simulink library "MofNFilterBlock"  (R2018b)
settings: Solver=VariableStepAuto  StartTime=0.0  StopTime=10.0  RelTol=1e-3
undefined symbols (not defined in the file): filter_M_down, filter_M_up, filter_N
libraries: simulink x1
settings Model: Creator=BI28030  LastModifiedBy=BI28030

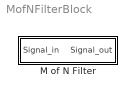
== system MofNFilterBlock ==
  M of N Filter : Subsystem  mask{num_samples=filter_N, num_upgrade=filter_M_up, num_downgrade=filter_M_down}
      mask prompts: num_samples "Number of Samples (N)"; num_upgrade "Number for Upgrade (M)"; num_downgrade "Number for Downgrade (M)"

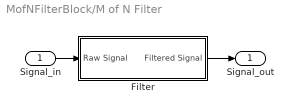
== system MofNFilterBlock/M of N Filter ==
  Signal_in : Inport
  Filter : Subsystem  mask(Alert Filter){num_samples_signal=num_samples, threshold_signal=num_upgrade, threshold_downgrade=num_downgrade}
      mask prompts: num_samples_signal "Number of Raw Signal Samples"; threshold_signal "Number of Positives for Signal upgrade"; threshold_downgrade "Number of Negatives for Downgrade"
      mask help: Filters stream of raw alerts to compensate for surveillance noise.
  Signal_out : Outport
  wires:
  Filter/1(Filtered Signal) -> Signal_out/1
  Signal_in/1 -> Filter/1(Raw Signal)

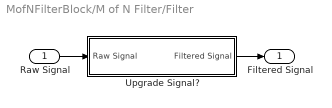
== system MofNFilterBlock/M of N Filter/Filter ==
  Raw Signal : Inport
  Upgrade Signal? : Subsystem  TreatAsAtomicUnit=on
  Filtered Signal : Outport
  wires:
  Upgrade Signal?/1(Filtered Signal) -> Filtered Signal/1
  Raw Signal/1 -> Upgrade Signal?/1(Raw Signal)

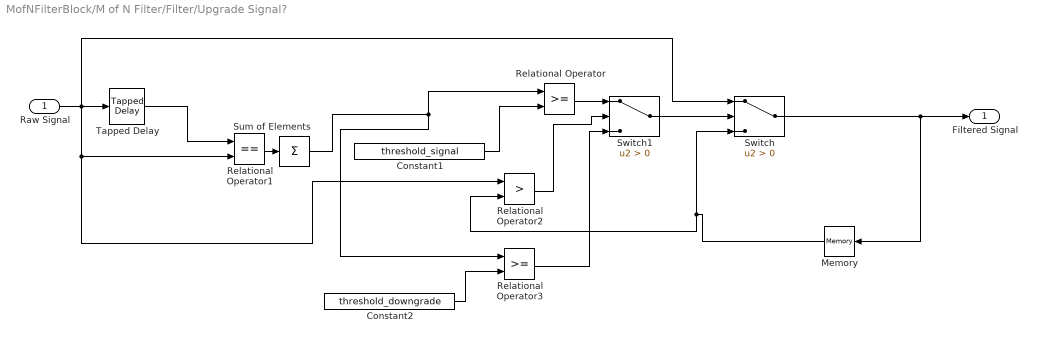
== system MofNFilterBlock/M of N Filter/Filter/Upgrade Signal? ==
  Raw Signal : Inport
  Constant1 : Constant  Value=threshold_signal
  Constant2 : Constant  Value=threshold_downgrade
  Memory : Memory  InheritSampleTime=on
  Relational Operator1 : RelationalOperator  Operator===  OutDataTypeStr=boolean  RndMeth=Simplest
  Relational Operator : RelationalOperator  OutDataTypeStr=boolean  RndMeth=Nearest
  Relational Operator2 : RelationalOperator  Operator=>  OutDataTypeStr=boolean  RndMeth=Nearest
  Relational Operator3 : RelationalOperator  OutDataTypeStr=boolean  RndMeth=Nearest
  Sum of Elements : Sum  Inputs=+
  Switch : Switch  Criteria=u2 > Threshold
  Switch1 : Switch  Criteria=u2 > Threshold
  Tapped Delay : simulink/Discrete/Tapped Delay  vinit=0.0  samptime=-1  NumDelays=num_samples_signal-1  DelayOrder=Oldest  includeCurrent=on
  Filtered Signal : Outport
  wires:
  Constant2/1 -> Relational Operator3/2
  Relational Operator3/1 -> Switch1/3
  Switch1/1 -> Switch/2
  Relational Operator2/1 -> Switch1/2
  Relational Operator1/1 -> Sum of Elements/1
  Sum of Elements/1 -> Relational Operator3/1, Relational Operator/1
  Constant1/1 -> Relational Operator/2
  Relational Operator/1 -> Switch1/1
  Raw Signal/1 -> Relational Operator1/2, Relational Operator2/1, Switch/1, Tapped Delay/1
  Tapped Delay/1 -> Relational Operator1/1
  Memory/1 -> Switch/3, Relational Operator2/2
  Switch/1 -> Memory/1, Filtered Signal/1
